simulink model "test"  (R2018a)
settings: Solver=VariableStepAuto  StartTime=0.0  StopTime=1  RelTol=1e-3
undefined symbols (not defined in the file): fdesignblkfcn, G1, G2, G3, G4, G5, G6, G7, G8, gcbh, get, T
libraries: dspsrcs4 x9, dspxfrm3 x2, dspobslib x2
(part 1 of 3)
settings Model: Creator=Daniel  LastModifiedBy=Daniel

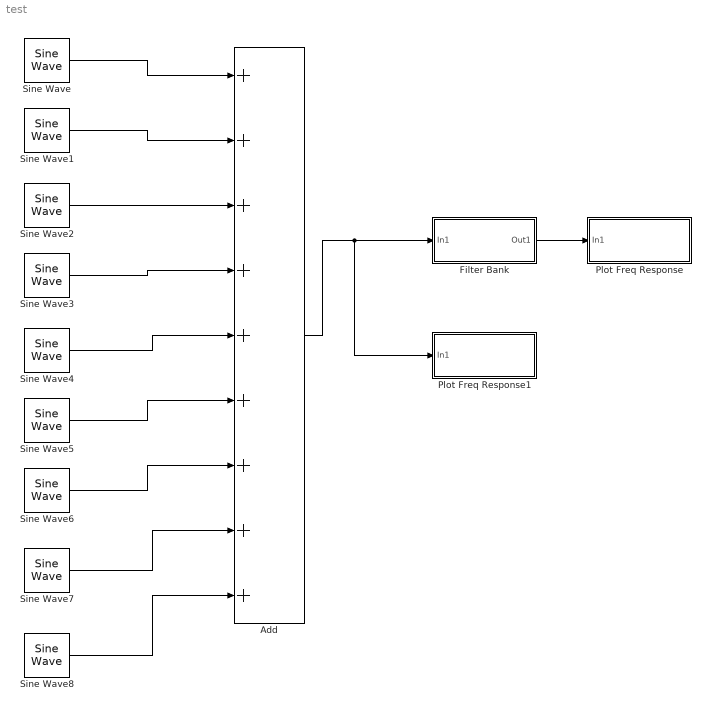
== system test ==
  Add : Sum  Inputs=+++++++++
  "Filter Bank " : Subsystem
  Plot Freq Response : Subsystem
  Plot Freq Response1 : Subsystem
  Sine Wave : dspsrcs4/Sine Wave  Amplitude=1  Frequency=500  Phase=0  SampleMode=Discrete  OutComplex=Real  CompMethod=Trigonometric fcn  TableSize=Speed  SampleTime=T  SamplesPerFrame=128  ResetState=Restart at time zero  OutputFrames=off  dataType=double  wordLen=16  udDataType=sfix(16)  fracBitsMode=Best precision  numFracBits=15  OutDataTypeStr=double  LastOutDataTypeStr=double
  Sine Wave1 : dspsrcs4/Sine Wave  Amplitude=1  Frequency=750  Phase=0  SampleMode=Discrete  OutComplex=Real  CompMethod=Trigonometric fcn  TableSize=Speed  SampleTime=T  SamplesPerFrame=128  ResetState=Restart at time zero  OutputFrames=off  dataType=double  wordLen=16  udDataType=sfix(16)  fracBitsMode=Best precision  numFracBits=15  OutDataTypeStr=double  LastOutDataTypeStr=double
  Sine Wave2 : dspsrcs4/Sine Wave  Amplitude=1  Frequency=1000  Phase=0  SampleMode=Discrete  OutComplex=Real  CompMethod=Trigonometric fcn  TableSize=Speed  SampleTime=T  SamplesPerFrame=128  ResetState=Restart at time zero  OutputFrames=off  dataType=double  wordLen=16  udDataType=sfix(16)  fracBitsMode=Best precision  numFracBits=15  OutDataTypeStr=double  LastOutDataTypeStr=double
  Sine Wave3 : dspsrcs4/Sine Wave  Amplitude=1  Frequency=1500  Phase=0  SampleMode=Discrete  OutComplex=Real  CompMethod=Trigonometric fcn  TableSize=Speed  SampleTime=T  SamplesPerFrame=128  ResetState=Restart at time zero  OutputFrames=off  dataType=double  wordLen=16  udDataType=sfix(16)  fracBitsMode=Best precision  numFracBits=15  OutDataTypeStr=double  LastOutDataTypeStr=double
  Sine Wave4 : dspsrcs4/Sine Wave  Amplitude=1  Frequency=2000  Phase=0  SampleMode=Discrete  OutComplex=Real  CompMethod=Trigonometric fcn  TableSize=Speed  SampleTime=T  SamplesPerFrame=128  ResetState=Restart at time zero  OutputFrames=off  dataType=double  wordLen=16  udDataType=sfix(16)  fracBitsMode=Best precision  numFracBits=15  OutDataTypeStr=double  LastOutDataTypeStr=double
  Sine Wave5 : dspsrcs4/Sine Wave  Amplitude=1  Frequency=2500  Phase=0  SampleMode=Discrete  OutComplex=Real  CompMethod=Trigonometric fcn  TableSize=Speed  SampleTime=T  SamplesPerFrame=128  ResetState=Restart at time zero  OutputFrames=off  dataType=double  wordLen=16  udDataType=sfix(16)  fracBitsMode=Best precision  numFracBits=15  OutDataTypeStr=double  LastOutDataTypeStr=double
  Sine Wave6 : dspsrcs4/Sine Wave  Amplitude=1  Frequency=3000  Phase=0  SampleMode=Discrete  OutComplex=Real  CompMethod=Trigonometric fcn  TableSize=Speed  SampleTime=T  SamplesPerFrame=128  ResetState=Restart at time zero  OutputFrames=off  dataType=double  wordLen=16  udDataType=sfix(16)  fracBitsMode=Best precision  numFracBits=15  OutDataTypeStr=double  LastOutDataTypeStr=double
  Sine Wave7 : dspsrcs4/Sine Wave  Amplitude=1  Frequency=3500  Phase=0  SampleMode=Discrete  OutComplex=Real  CompMethod=Trigonometric fcn  TableSize=Speed  SampleTime=T  SamplesPerFrame=128  ResetState=Restart at time zero  OutputFrames=off  dataType=double  wordLen=16  udDataType=sfix(16)  fracBitsMode=Best precision  numFracBits=15  OutDataTypeStr=double  LastOutDataTypeStr=double
  Sine Wave8 : dspsrcs4/Sine Wave  Amplitude=1  Frequency=4000  Phase=0  SampleMode=Discrete  OutComplex=Real  CompMethod=Trigonometric fcn  TableSize=Speed  SampleTime=T  SamplesPerFrame=128  ResetState=Restart at time zero  OutputFrames=off  dataType=double  wordLen=16  udDataType=sfix(16)  fracBitsMode=Best precision  numFracBits=15  OutDataTypeStr=double  LastOutDataTypeStr=double
  wires:
  "Filter Bank "/1(Out1) -> Plot Freq Response/1(In1)
  Add/1 -> Plot Freq Response1/1(In1), "Filter Bank "/1(In1)
  Sine Wave/1 -> Add/1
  Sine Wave1/1 -> Add/2
  Sine Wave2/1 -> Add/3
  Sine Wave3/1 -> Add/4
  Sine Wave4/1 -> Add/5
  Sine Wave5/1 -> Add/6
  Sine Wave6/1 -> Add/7
  Sine Wave7/1 -> Add/8
  Sine Wave8/1 -> Add/9

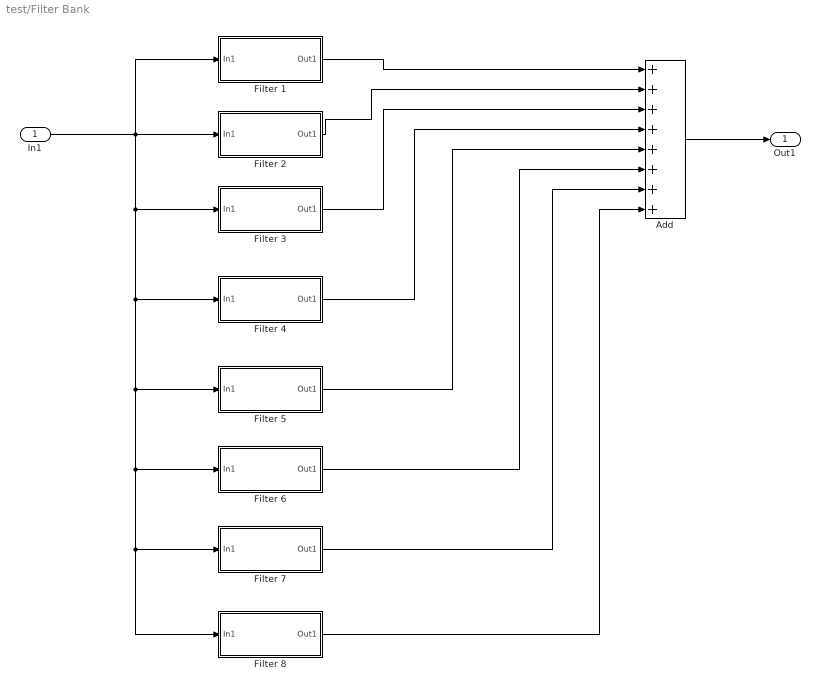
== system test/Filter Bank  ==
  In1 : Inport
  Add : Sum  Inputs=++++++++
  Filter 1 : Subsystem
  Filter 2 : Subsystem
  Filter 3 : Subsystem
  Filter 4 : Subsystem
  Filter 5 : Subsystem
  Filter 6 : Subsystem
  Filter 7 : Subsystem
  Filter 8 : Subsystem
  Out1 : Outport
  wires:
  In1/1 -> Filter 6/1(In1), Filter 8/1(In1), Filter 7/1(In1), Filter 5/1(In1), Filter 4/1(In1), Filter 3/1(In1), Filter 1/1(In1), Filter 2/1(In1)
  Add/1 -> Out1/1
  Filter 1/1(Out1) -> Add/1
  Filter 2/1(Out1) -> Add/2
  Filter 3/1(Out1) -> Add/3
  Filter 4/1(Out1) -> Add/4
  Filter 5/1(Out1) -> Add/5
  Filter 6/1(Out1) -> Add/6
  Filter 7/1(Out1) -> Add/7
  Filter 8/1(Out1) -> Add/8

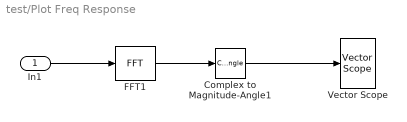
== system test/Plot Freq Response ==
  In1 : Inport
  Complex to Magnitude-Angle1 : ComplexToMagnitudeAngle  Output=Magnitude
  FFT1 : dspxfrm3/FFT  FFTImplementation=Auto  CompMethod=Table lookup  TableOpt=NEW  TableOptActive=Speed  BitRevOrder=off  Normalize=off  InheritFFTLength=on  FFTLength=64  WrapInput=on  roundingMode=Floor  overflowMode=off  firstCoeffDataTypeStr=Inherit: Same word length as input  firstCoeffLastDataTypeStr=Inherit: Same word length as input  outputMin=[]  outputMax=[]
  Vector Scope : dspobslib/Vector Scope  ScopeProperties=off  Domain=Frequency  HorizSpan=1  DisplayProperties=off  AxisGrid=on  Memory=off  FrameNumber=off  AxisLegend=off  AxisZoom=off  OpenScopeAtSimStart=on  OpenScopeImmediately=off  FigPos=get(0,'defaultfigureposition')  AxisProperties=on  XUnits=Hertz  XRange=[0...Fs/2]  InheritXIncr=on  XIncr=1  XLabel=Samples  XLimit=Auto  XMin=0  XMax=1  XStart=0  YUnits=dB  YLabel=|Magnitude (dB)|  LineProperties=off  XAxisParamsVer=6.9
      settings: SourceProductName=DSP System Toolbox  SourceProductBaseCode=DS  YMin=0.0723692553519949  YMax=69.3188381671759
  wires:
  In1/1 -> FFT1/1
  FFT1/1 -> Complex to Magnitude-Angle1/1
  Complex to Magnitude-Angle1/1 -> Vector Scope/1

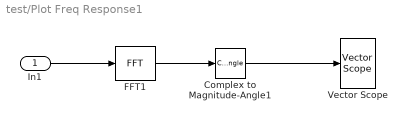
== system test/Plot Freq Response1 ==
  In1 : Inport
  Complex to Magnitude-Angle1 : ComplexToMagnitudeAngle  Output=Magnitude
  FFT1 : dspxfrm3/FFT  FFTImplementation=Auto  CompMethod=Table lookup  TableOpt=NEW  TableOptActive=Speed  BitRevOrder=off  Normalize=off  InheritFFTLength=on  FFTLength=64  WrapInput=on  roundingMode=Floor  overflowMode=off  firstCoeffDataTypeStr=Inherit: Same word length as input  firstCoeffLastDataTypeStr=Inherit: Same word length as input  outputMin=[]  outputMax=[]
  Vector Scope : dspobslib/Vector Scope  ScopeProperties=off  Domain=Frequency  HorizSpan=1  DisplayProperties=off  AxisGrid=on  Memory=off  FrameNumber=off  AxisLegend=off  AxisZoom=off  OpenScopeAtSimStart=on  OpenScopeImmediately=off  FigPos=get(0,'defaultfigureposition')  AxisProperties=on  XUnits=Hertz  XRange=[0...Fs/2]  InheritXIncr=on  XIncr=1  XLabel=Samples  XLimit=Auto  XMin=0  XMax=1  XStart=0  YUnits=dB  YLabel=|Magnitude (dB)|  LineProperties=off  XAxisParamsVer=6.9
      settings: SourceProductName=DSP System Toolbox  SourceProductBaseCode=DS  YMin=0.0723692553519949  YMax=69.3188381671759
  wires:
  In1/1 -> FFT1/1
  FFT1/1 -> Complex to Magnitude-Angle1/1
  Complex to Magnitude-Angle1/1 -> Vector Scope/1

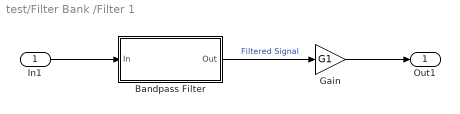
== system test/Filter Bank /Filter 1 ==
  In1 : Inport
  Bandpass Filter : Subsystem  DialogController=fdesignblkfcn  InitFcn=fdesignblkfcn(gcbh, {'InitFcn'});  mask(Bandpass Filter){}
      mask help: Design a bandpass filter
      settings: CopyFcn=fdesignblkfcn(gcbh, {'CopyFcn'});
      mask Help: helpview(mapfilelocation('dsp'), 'dspbandpassfilter');
      mask Display: disp('Bandpass');
  Gain : Gain  Gain=G1
  Out1 : Outport
  wires:
  Bandpass Filter/1(Out) -> Gain/1  "Filtered Signal"
  In1/1 -> Bandpass Filter/1(In)
  Gain/1 -> Out1/1

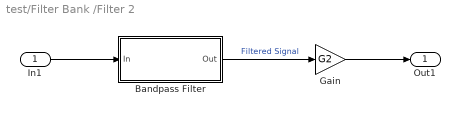
== system test/Filter Bank /Filter 2 ==
  In1 : Inport
  Bandpass Filter : Subsystem  DialogController=fdesignblkfcn  InitFcn=fdesignblkfcn(gcbh, {'InitFcn'});  mask(Bandpass Filter){}
      mask help: Design a bandpass filter
      settings: CopyFcn=fdesignblkfcn(gcbh, {'CopyFcn'});
      mask Help: helpview(mapfilelocation('dsp'), 'dspbandpassfilter');
      mask Display: disp('Bandpass');
  Gain : Gain  Gain=G2
  Out1 : Outport
  wires:
  Bandpass Filter/1(Out) -> Gain/1  "Filtered Signal"
  In1/1 -> Bandpass Filter/1(In)
  Gain/1 -> Out1/1

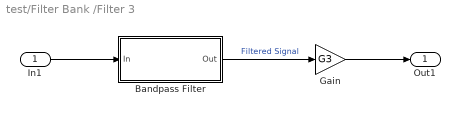
== system test/Filter Bank /Filter 3 ==
  In1 : Inport
  Bandpass Filter : Subsystem  DialogController=fdesignblkfcn  InitFcn=fdesignblkfcn(gcbh, {'InitFcn'});  mask(Bandpass Filter){}
      mask help: Design a bandpass filter
      settings: CopyFcn=fdesignblkfcn(gcbh, {'CopyFcn'});
      mask Help: helpview(mapfilelocation('dsp'), 'dspbandpassfilter');
      mask Display: disp('Bandpass');
  Gain : Gain  Gain=G3
  Out1 : Outport
  wires:
  Bandpass Filter/1(Out) -> Gain/1  "Filtered Signal"
  In1/1 -> Bandpass Filter/1(In)
  Gain/1 -> Out1/1

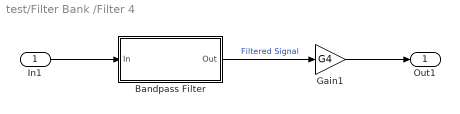
== system test/Filter Bank /Filter 4 ==
  In1 : Inport
  Bandpass Filter : Subsystem  DialogController=fdesignblkfcn  InitFcn=fdesignblkfcn(gcbh, {'InitFcn'});  mask(Bandpass Filter){}
      mask help: Design a bandpass filter
      settings: CopyFcn=fdesignblkfcn(gcbh, {'CopyFcn'});
      mask Help: helpview(mapfilelocation('dsp'), 'dspbandpassfilter');
      mask Display: disp('Bandpass');
  Gain1 : Gain  Gain=G4
  Out1 : Outport
  wires:
  Bandpass Filter/1(Out) -> Gain1/1  "Filtered Signal"
  In1/1 -> Bandpass Filter/1(In)
  Gain1/1 -> Out1/1

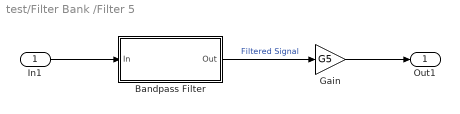
== system test/Filter Bank /Filter 5 ==
  In1 : Inport
  Bandpass Filter : Subsystem  DialogController=fdesignblkfcn  InitFcn=fdesignblkfcn(gcbh, {'InitFcn'});  mask(Bandpass Filter){}
      mask help: Design a bandpass filter
      settings: CopyFcn=fdesignblkfcn(gcbh, {'CopyFcn'});
      mask Help: helpview(mapfilelocation('dsp'), 'dspbandpassfilter');
      mask Display: disp('Bandpass');
  Gain : Gain  Gain=G5
  Out1 : Outport
  wires:
  Bandpass Filter/1(Out) -> Gain/1  "Filtered Signal"
  In1/1 -> Bandpass Filter/1(In)
  Gain/1 -> Out1/1

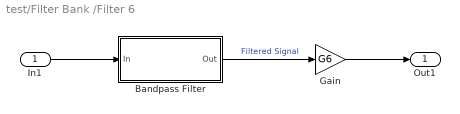
== system test/Filter Bank /Filter 6 ==
  In1 : Inport
  Bandpass Filter : Subsystem  DialogController=fdesignblkfcn  InitFcn=fdesignblkfcn(gcbh, {'InitFcn'});  mask(Bandpass Filter){}
      mask help: Design a bandpass filter
      settings: CopyFcn=fdesignblkfcn(gcbh, {'CopyFcn'});
      mask Help: helpview(mapfilelocation('dsp'), 'dspbandpassfilter');
      mask Display: disp('Bandpass');
  Gain : Gain  Gain=G6
  Out1 : Outport
  wires:
  Bandpass Filter/1(Out) -> Gain/1  "Filtered Signal"
  In1/1 -> Bandpass Filter/1(In)
  Gain/1 -> Out1/1

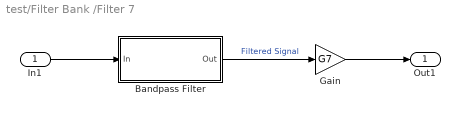
== system test/Filter Bank /Filter 7 ==
  In1 : Inport
  Bandpass Filter : Subsystem  DialogController=fdesignblkfcn  InitFcn=fdesignblkfcn(gcbh, {'InitFcn'});  mask(Bandpass Filter){}
      mask help: Design a bandpass filter
      settings: CopyFcn=fdesignblkfcn(gcbh, {'CopyFcn'});
      mask Help: helpview(mapfilelocation('dsp'), 'dspbandpassfilter');
      mask Display: disp('Bandpass');
  Gain : Gain  Gain=G7
  Out1 : Outport
  wires:
  Bandpass Filter/1(Out) -> Gain/1  "Filtered Signal"
  In1/1 -> Bandpass Filter/1(In)
  Gain/1 -> Out1/1

== system test/Filter Bank /Filter 8 ==
  In1 : Inport
  Bandpass Filter : Subsystem  DialogController=fdesignblkfcn  InitFcn=fdesignblkfcn(gcbh, {'InitFcn'});  mask(Bandpass Filter){}
      mask help: Design a bandpass filter
      settings: CopyFcn=fdesignblkfcn(gcbh, {'CopyFcn'});
      mask Help: helpview(mapfilelocation('dsp'), 'dspbandpassfilter');
      mask Display: disp('Bandpass');
  Gain : Gain  Gain=G8
  Out1 : Outport
  wires:
  Bandpass Filter/1(Out) -> Gain/1  "Filtered Signal"
  In1/1 -> Bandpass Filter/1(In)
  Gain/1 -> Out1/1

== system test/Filter Bank /Filter 1/Bandpass Filter ==
  In : Inport
  Generated Filter Block : DiscreteFir  Tag=BlockMethodSubSystem  Coefficients=[0.00099033939918158711 7.84794241453230898e-05 8.12930927527524279e-05 8.38881428959181686e-05 8.63707452084759293e-05 8.85902365413272872e-05 9.06595221473260415e-05 9.2431230842850799e-05 9.4015690076486175e-05 9.52611340743902702e-05 9.62914005701961164e-05 9.69492456172241197e-05 9.73637356417781074e-05 9.73797400380331768e-05 9.71507038179902064e-05 9.65155801599824263e-05 9.56410785019714448e-05 9.43615771392707818e-05 9.28723174557975854e-05 9.09860962634488716e-05 8.89093706643017138e-05 8.64199507881054606e-05 8.3748969405348785e-05 8.06140130326997542e-05 7.72702456115150372e-05 7.33659635393778151e-05 6.92536876552578729e-05 6.45259894628607086e-05 5.98133168057183079e-05 5.47025680392715166e-05 5.05355035232757713e-05 4.60457931258272861e-05 3.87270014004957645e-05 3.40808925056528781e-05 2.79786361072961895e-05 2.22818921811813086e-05 1.61514077488016877e-05 1.0244378171210493e-05 4.10156392738902693e-06 -1.82851402803579054e-06 -7.85932539815617794e-06 -1.36325002849443842e-05 -1.939813580992241e-05 -2.48557609549429769e-05 -3.02048320336083667e-05 -3.51760945588823815e-05 -3.99491232367016932e-05 -4.4274621620911419e-05 -4.83003717722137781e-05 -5.17765808001552372e-05 -5.48393887127774756e-05 -5.72395293973769885e-05 -5.91019783105518271e-05 -6.01790684081319297e-05 -6.06268751331873984e-05 -6.02178253312065314e-05 -5.91453808850374825e-05 -5.71590475185277338e-05 -5.44489729162290915e-05 -5.06109018152955337e-05 -4.58139883559535133e-05 -3.95713158674203521e-05 -3.27868034529527701e-05 -2.49402282669318848e-05 -1.53345720735928455e-05 -5.03237188454855924e-06 6.78816683646451716e-06 1.97214774302365836e-05 3.40697878597185207e-05 4.96538003962004561e-05 6.66567029871035404e-05 8.49746685666716051e-05 0.000104736051705015521 0.000125854597006872952 0.000148431089153642153 0.000172396191630700275 0.000197818727877812191 0.000224617994448285039 0.000252845875461143706 0.000282425796709244578 0.000313395957969779082 0.000345672795687264659 0.000379297150580223757 0.000414190646573953818 0.000450383663613797161 0.000487762395661845609 0.00052632855538739488 0.000565930108540442988 0.00060657134029451856 0.000648117161834510232 0.000690657965575478742 0.000734022224926053559 0.000778206743131040464 0.00082272462701590051 0.000868031974373832389 0.000913839077680649297 0.000959813439322741496 0.00100618519857815906 0.00105258004367821795 0.00109905367823569201 0.0011453419108028906 0.00119142711097145393 0.00123708687606507431 0.00128225804862928104 0.00132672980218272001 0.00137043172498172794 0.00141316065858932598 0.00145481907415349605 0.00149519812702366144 0.00153419419216097941 0.00157159674549731837 0.00160728617361893507 0.00164105341897468325 0.00167279337441302869 0.00170231045121560878 0.00172949478173076176 0.0017541347802007641 0.00177610605222130622 0.00179518410354805383 0.00181126402258718682 0.00182416489466682183 0.00183382737651553046 0.00184001381449865986 0.00184258175116447766 0.00184127385668097295 0.00183629223891175215 0.00182716391605073606 0.00181389928125657153 0.00179641258380717822 0.00177451504550320011 0.00174815685808793128 0.00171719084373056388 0.00168156279041510527 0.00164115693412843189 0.00159590832620988207 0.00154573841173723161 0.00149060801525829011 0.00143045805685813074 0.0013652560796938698 0.00129497061950771129 0.00121959218680503544 0.00113910233009925513 0.00105350082094989896 0.000962800176844101196 0.000867039733145126752 0.000766262863169200913 0.00066052533090125206 0.000549882617799260552 0.0004344024324556683 0.000314162090958703072 0.000189279222698524675 5.98905940741293851e-05 -7.38666451062696327e-05 -0.000211897796086117174 -0.000354075089992386346 -0.000500193210865189472 -0.000649982139995642695 -0.000803466607903623349 -0.000960259479657047895 -0.00112022533600402178 -0.00128312683678756664 -0.00144871991890352272 -0.00161676554861868048 -0.00178698607972570191 -0.001959137417076848 -0.00213293099453609096 -0.00230808256105186939 ...(+9428 chars)]  InputProcessing=Columns as channels (frame based)
  Out : Outport
  wires:
  In/1 -> Generated Filter Block/1
  Generated Filter Block/1 -> Out/1

== system test/Filter Bank /Filter 2/Bandpass Filter ==
  In : Inport
  Generated Filter Block : Subsystem  Tag=FilterWizardSubSystem
      settings: ErrorFcn=dspFilterRealizedInBasicElemsAlgLoopErrFcnCallback
  Out : Outport
  wires:
  In/1 -> Generated Filter Block/1(Input)
  Generated Filter Block/1(Output) -> Out/1

== system test/Filter Bank /Filter 3/Bandpass Filter ==
  In : Inport
  Generated Filter Block : DiscreteFir  Tag=BlockMethodSubSystem  Coefficients=[-0.000562669441124423572 -0.000176319248460171576 -0.000201252087180046836 -0.000226545778209361325 -0.000251654091483891236 -0.000276242966267669884 -0.000299683484186093316 -0.000321599476008826209 -0.00034133027166279343 -0.00035849719216703472 -0.000372442556913966992 -0.000382789226616923601 -0.000388861691491732095 -0.000390270637747746393 -0.000386325995989758141 -0.000376688953076411489 -0.0003607526372122188 -0.000338371437030749931 -0.000309125555400756736 -0.000273067800563625855 -0.000229853188865842233 -0.000179588241972150381 -0.00012195190324706716 -5.73513460211483054e-05 1.4089114910176977e-05 9.13412180418954437e-05 0.000174361216098270646 0.000262528186275067085 0.000356195843986883542 0.000452029942155993255 0.000551279587941525765 0.00065238344118258827 0.000753562081010308968 0.000854535536502646687 0.000953348741316194974 0.00104924403516426772 0.00114049293461653011 0.00122607681334865014 0.00130435438702659542 0.00137422661632990084 0.00143418540367142976 0.00148321240171634663 0.00152000245324606558 0.00154367997325479452 0.00155312806667693218 0.00154765713165035774 0.00152644723908830298 0.00148916530443843082 0.00143541786351509865 0.00136521786952889892 0.00127846281105446964 0.00117548230837075931 0.00105666328730298154 0.000922937118449187934 0.000775060071358566458 0.000614137560950027807 0.00044130413461738766 0.000258538967978680281 6.70705572613053717e-05 -0.000131270118101637636 -0.000334171925003715899 -0.000540008689574483693 -0.00074624536606872024 -0.000950878407127821309 -0.00115150100877486807 -0.00134594610525745053 -0.00153191134765045004 -0.00170725255233676555 -0.00186980828902552805 -0.002017609672253751 -0.00214878948321399173 -0.00226172364662780056 -0.00235493555882275224 -0.0024272008505058576 -0.00247748951856042489 -0.00250508491799861406 -0.00250956240989992727 -0.00249080295772724112 -0.00244894606056840535 -0.00238442917286214385 -0.00229803976196877365 -0.00219091711863159859 -0.00206439991183875833 -0.00192007331986474949 -0.00175985962897826759 -0.00158600584074588039 -0.0014007690106329798 -0.00120661552841093227 -0.00100643714049005058 -0.000802722303215981149 -0.000598515192319599033 -0.000396560067281224277 -0.00019974287848621342 -1.0828883101161039e-05 0.000167544906071088513 0.000332872424030146723 0.00048286562104317448 0.00061543992373154781 0.000728815751403747011 0.000821508163233834851 0.000892403535207162389 0.000940725603427471405 0.000966101116937096859 0.000968536338935308623 0.000948513408730399898 0.000906888944684994952 0.000844953212706004353 0.000764349027059558258 0.000667186188656383543 0.000555936287401684521 0.000433385274901638615 0.000302580973515108635 0.000166916729102523689 2.99709377234033954e-05 -0.000104544428638633181 -0.000232827460083235709 -0.000350856143596712405 -0.000454908372407157537 -0.000541083925529831848 -0.00060577222949807579 -0.000645546111373450707 -0.000657188177991202896 -0.000637920072851291126 -0.000585268607311083592 -0.000497288253651437121 -0.000372473795498794939 -0.000209917224807805837 -9.26387264281570714e-06 0.00022918023961401469 0.000504501276895290523 0.000815112434008402457 0.00115879264957740365 0.00153260742325761088 0.00193300664120614604 0.00235580853290004227 0.00279627618639841785 0.00324909117034294934 0.00370843180457892854 0.00416808412821790056 0.00462146051745883357 0.00506165836813182463 0.00548159619960417697 0.00587410097134965104 0.006231976924177169 0.00654804415861365719 0.00681542417028926754 0.00702742438742094255 0.00717776202446580511 0.00726069908607346066 0.00727095543981547653 0.00720406654629939143 0.0070562064724531727 0.00682447697331475464 0.00650681992220087605 0.00610218661268093366 0.00561051159729753727 0.00503282623705536732 0.00437121583448081292 0.00362887039672928416 0.00281004232086383421 0.00192010113860904656 0.000965442550076401913 -4.65296364593799716e-05 -0.00110747884426670262 -0.00220817944630956721 -0.00333859815816218205 -0.00448805226743928531 ...(+6161 chars)]  InputProcessing=Columns as channels (frame based)
  Out : Outport
  wires:
  In/1 -> Generated Filter Block/1
  Generated Filter Block/1 -> Out/1

== system test/Filter Bank /Filter 4/Bandpass Filter ==
  In : Inport
  Generated Filter Block : DiscreteFir  Tag=BlockMethodSubSystem  Coefficients=[0.000627119134687924209 0.000344548775358714593 0.00042484106297373714 0.000506484659751256418 0.000585861666298503805 0.000659108756263350492 0.000720998715683666557 0.000767569078092942983 0.000794450476974133081 0.000797734151546513432 0.000771611723369832847 0.00071528375080963998 0.000624966668657625491 0.000499181040108482633 0.000338342763470004062 0.000142556867295336035 -8.46743014055733744e-05 -0.000339746401218691987 -0.000616952448113500555 -0.000909913232528025738 -0.00121002835462913653 -0.00150887164410737178 -0.00179656089414822334 -0.00206293679049682991 -0.00229821459579304405 -0.0024922416585774973 -0.00263635114058083202 -0.00272283331458696414 -0.0027455746492955819 -0.00270036903867938022 -0.00258533226333800556 -0.00240091253505882824 -0.00215006525718239739 -0.00183858721182439356 -0.00147426241973875769 -0.00106775293822941012 -0.000631331238739624157 -0.000178975931644154184 0.000274241695372509945 0.000712763571602798235 0.00112114852533595484 0.00148473702670122768 0.00179032134207000372 0.00202698151632994946 0.00218625655690362578 0.00226313994956952712 0.00225619234773988351 0.00216779013786963688 0.00200447899729562333 0.00177659634554368619 0.00149833509456900752 0.00118715735301868101 0.00086335288419918106 0.00054905680419437301 0.000267697031500487828 4.2716988300645466e-05 -0.000103368547561563694 -0.000150000144935029704 -7.98842308931896686e-05 0.000120225192370502132 0.000458437493729260237 0.000936976644482716823 0.0015515853477789136 0.00229121185785128526 0.0031378161670221295 0.00406656740504704635 0.00504635039897608113 0.0060403018958571416 0.00700709471698401747 0.00790195448977607309 0.00867826171340673608 0.00928918788171108518 0.00968945953566448595 0.0098371784944074718 0.00969567432215362457 0.0092352360414894516 0.00843465921243507881 0.00728277995918044825 0.00577940780164222165 0.00393621520208512106 0.00177713536991783942 -0.000661720009975110663 -0.00333239894016079067 -0.00617605137205823156 -0.00912418581865912133 -0.0121003887284758891 -0.015022285346619025 -0.0178040206245435872 -0.0203586932223662823 -0.0226011378172533209 -0.0244507212202955092 -0.0258339975460141098 -0.0266874206108171919 -0.0269596795469024125 -0.0266137900699570593 -0.0256287856113014828 -0.0240009935502928026 -0.0217446801986343752 -0.0188922837533984783 -0.0154940088142689631 -0.0116167886360870644 -0.0073428835998597293 -0.00276773320968613876 0.00200248051706282187 0.00685371479326360358 0.0116672407015916586 0.0163230416545682294 0.0207032251013506974 0.0246955062027547703 0.0281965336362828486 0.0311148882541423602 0.0333739403785469207 0.0349140647535569337 0.0356944746398965562 0.0356944746398965562 0.0349140647535569337 0.0333739403785469207 0.0311148882541423602 0.0281965336362828486 0.0246955062027547703 0.0207032251013506974 0.0163230416545682294 0.0116672407015916586 0.00685371479326360358 0.00200248051706282187 -0.00276773320968613876 -0.0073428835998597293 -0.0116167886360870644 -0.0154940088142689631 -0.0188922837533984783 -0.0217446801986343752 -0.0240009935502928026 -0.0256287856113014828 -0.0266137900699570593 -0.0269596795469024125 -0.0266874206108171919 -0.0258339975460141098 -0.0244507212202955092 -0.0226011378172533209 -0.0203586932223662823 -0.0178040206245435872 -0.015022285346619025 -0.0121003887284758891 -0.00912418581865912133 -0.00617605137205823156 -0.00333239894016079067 -0.000661720009975110663 0.00177713536991783942 0.00393621520208512106 0.00577940780164222165 0.00728277995918044825 0.00843465921243507881 0.0092352360414894516 0.00969567432215362457 0.0098371784944074718 0.00968945953566448595 0.00928918788171108518 0.00867826171340673608 0.00790195448977607309 0.00700709471698401747 0.0060403018958571416 0.00504635039897608113 0.00406656740504704635 0.0031378161670221295 0.00229121185785128526 0.0015515853477789136 0.000936976644482716823 0.000458437493729260237 0.000120225192370502132 -7.98842308931896686e-05 -0.000150000144935029704 -0.000103368547561563694 ...(+1331 chars)]  InputProcessing=Columns as channels (frame based)
  Out : Outport
  wires:
  In/1 -> Generated Filter Block/1
  Generated Filter Block/1 -> Out/1

== system test/Filter Bank /Filter 5/Bandpass Filter ==
  In : Inport
  Generated Filter Block : DiscreteFir  Tag=BlockMethodSubSystem  Coefficients=[-0.000409572521006904802 0.000169693844292237851 0.000199322260796864993 0.000251562507725645965 0.000310964698009966287 0.00036349141059103553 0.000396428874991713788 0.000400712250634985159 0.000371219716352128547 0.000308834019637180897 0.000219699661407548642 0.000115944018981461083 1.30065305809744236e-05 -7.12142161793231942e-05 -0.000120683673594628056 -0.000122538233013547583 -7.19845813252586899e-05 2.80901233503946064e-05 0.000162669559356228433 0.000309292560380890907 0.000436155587516622565 0.00050584550134297494 0.000485926647082892229 0.000346659449942015154 7.1539826698203187e-05 -0.000340311161486721715 -0.000869382307611035743 -0.00147669823367354907 -0.00210444192333373095 -0.00268183019212321454 -0.00313127630590003155 -0.00337836136868442573 -0.00336068557125264716 -0.00303803846942908573 -0.00239914555391560662 -0.00146721288077062686 -0.00029975904974555601 0.00101364205946320859 0.00236081799253273945 0.00361604810630734505 0.00465643355131799101 0.00537481571579634214 0.00569357639439798703 0.00557607274323906714 0.00503280519141101682 0.00412202894203549802 0.00294461021546900533 0.00163300762457970839 0.000335726604696662593 -0.000801326910739463003 -0.00165381347543665973 -0.00213624037172098404 -0.00221465680815588917 -0.00191334585784089478 -0.00131355415609902258 -0.00054474730576222223 0.000231616617319447947 0.00084348645864068322 0.0011321752668397916 0.000976932319665589589 0.000314130104093936083 -0.000848252824051354574 -0.00242620729522766143 -0.00426508286469654777 -0.00615516198497933261 -0.0078553941104552872 -0.00912345441513621319 -0.0097477509145120142 -0.00957774497812656153 -0.00854782857067377944 -0.00669179992090718125 -0.00414478870489467729 -0.00113220323912070786 0.00205432012879169226 0.00509060382940443746 0.00766047833194217348 0.00949689273868371472 0.0104195319371379776 0.0103623520488098624 0.00938757221524820842 0.00768346818004565085 0.00554437169306478631 0.00333532975475163982 0.00144473347040351748 0.000230522848840828396 -3.35872123419161473e-05 0.000795722832298267208 0.0026990963450923282 0.00548161263459895094 0.00878212584738162494 0.0121056251393921923 0.0148759046395198751 0.0165035904999389291 0.0164618081455700747 0.0143611514256746665 0.0100139157919359647 0.00347985339133290118 -0.00491448955362438003 -0.0145856598023444244 -0.0247345471205284752 -0.034415215062320155 -0.0426256506115775605 -0.0484108895673359962 -0.0509682246615059398 -0.0497420955791356006 -0.0444981452981606171 -0.0353669684330950307 -0.0228519037029677671 -0.0077981579043137645 0.00867436904920439351 0.0252689028092244264 0.0406302819515293387 0.0534727186644622238 0.0627030778380203158 0.0675271098489146904 0.0675271098489146904 0.0627030778380203158 0.0534727186644622238 0.0406302819515293387 0.0252689028092244264 0.00867436904920439351 -0.0077981579043137645 -0.0228519037029677671 -0.0353669684330950307 -0.0444981452981606171 -0.0497420955791356006 -0.0509682246615059398 -0.0484108895673359962 -0.0426256506115775605 -0.034415215062320155 -0.0247345471205284752 -0.0145856598023444244 -0.00491448955362438003 0.00347985339133290118 0.0100139157919359647 0.0143611514256746665 0.0164618081455700747 0.0165035904999389291 0.0148759046395198751 0.0121056251393921923 0.00878212584738162494 0.00548161263459895094 0.0026990963450923282 0.000795722832298267208 -3.35872123419161473e-05 0.000230522848840828396 0.00144473347040351748 0.00333532975475163982 0.00554437169306478631 0.00768346818004565085 0.00938757221524820842 0.0103623520488098624 0.0104195319371379776 0.00949689273868371472 0.00766047833194217348 0.00509060382940443746 0.00205432012879169226 -0.00113220323912070786 -0.00414478870489467729 -0.00669179992090718125 -0.00854782857067377944 -0.00957774497812656153 -0.0097477509145120142 -0.00912345441513621319 -0.0078553941104552872 -0.00615516198497933261 -0.00426508286469654777 -0.00242620729522766143 -0.000848252824051354574 0.000314130104093936083 0.000976932319665589589 ...(+1407 chars)]  InputProcessing=Columns as channels (frame based)
  Out : Outport
  wires:
  In/1 -> Generated Filter Block/1
  Generated Filter Block/1 -> Out/1
